simulink library "protectionLib"  (R2026a)
settings: Solver=VariableStepAuto
undefined symbols (not defined in the file or in its folder): DiscIntNeverNeededParam
settings Model: Creator=smred  LastModifiedBy=smred

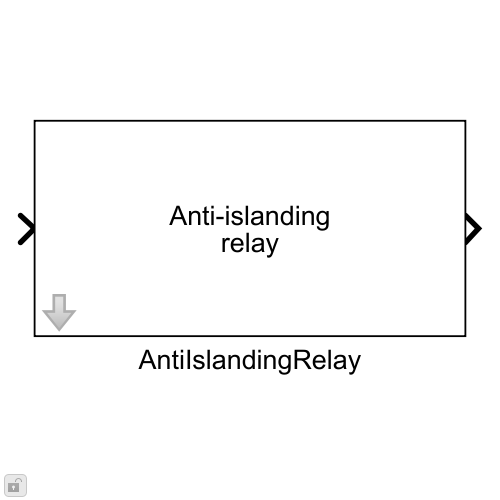
[thumbnail: Simulink's stored preview of the top-level diagram]
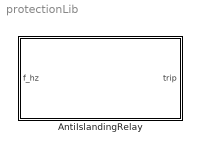
== system protectionLib ==
  AntiIslandingRelay : Subsystem  mask{f_min=47, f_max=52, t_arm=0.5, t_pickup=0.05, Ts=1e-4}
      mask prompts: f_min "Under-frequency trip (Hz)"; f_max "Over-frequency trip (Hz)"; t_arm "Relay blocked until (s)"; t_pickup "Out-of-band must persist (s)"; Ts "Persistence timer rate (s)"
      mask help:
      | Over/under-frequency relay with startup blocking and a persistence delay.
      |
      | Latches trip when the frequency estimate has been outside [f_min, f_max] continuously for t_pickup, and only after t_arm.
      |
      | BLOCKING (t_arm): a PLL frequency estimate is meaningless until the loop has acquired lock. Aqib's SRF-PLL leaves the 47-52 Hz band for up to 170 ms at startup, worst case at a 270 deg initial phase. Without blocking the relay latches at t = 0.
      |
      | PERSISTENCE (t_pickup): a 30 deg phase jump - the SC4 stimulus, which the PLL is specified to ride through - drives the estimate to 60 Hz for 12.4 ms, and a 60 deg jump for 20.7 ms. Without persistence the relay trips on a grid event the plant must survive. The default 50 ms gives 2.4x margin on the worst of those.
      |
      | Both figures are measured: see pll_startup_probe and pll_jump_probe.
      |
      | The latch is permanent. AS/NZS 4777.2 requires reconnection after 60 s within limits; that is not implemented here.
      mask Display: disp('Anti-islanding\nrelay')

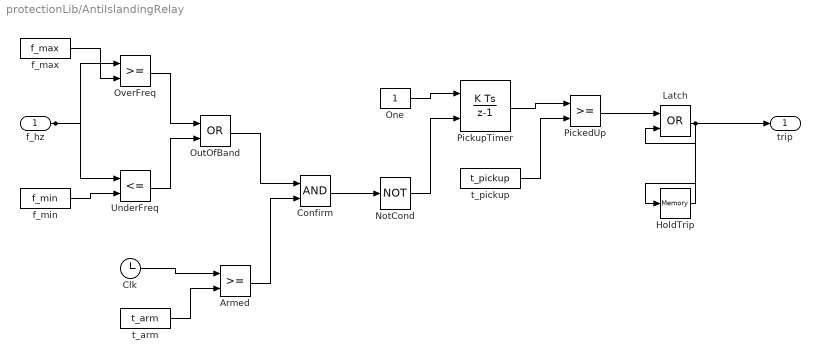
== system protectionLib/AntiIslandingRelay ==
  f_hz : Inport
  Armed : RelationalOperator  OutDataTypeStr=boolean  RndMeth=Simplest  InputSameDT=off
  Clk : Clock
  Confirm : Logic  AllPortsSameDT=off  OutDataTypeStr=boolean
  HoldTrip : Memory
  Latch : Logic  Operator=OR  AllPortsSameDT=off  OutDataTypeStr=boolean
  NotCond : Logic  Operator=NOT  Inputs=1  AllPortsSameDT=off  OutDataTypeStr=boolean
  One : Constant
  OutOfBand : Logic  Operator=OR  AllPortsSameDT=off  OutDataTypeStr=boolean
  OverFreq : RelationalOperator  OutDataTypeStr=boolean  RndMeth=Simplest  InputSameDT=off
  PickedUp : RelationalOperator  OutDataTypeStr=boolean  RndMeth=Simplest  InputSameDT=off
  PickupTimer : DiscreteIntegrator  gainval=1  ExternalReset=level  SampleTime=Ts  ICPrevOutput=DiscIntNeverNeededParam  ICPrevScaledInput=DiscIntNeverNeededParam
  UnderFreq : RelationalOperator  Operator=<=  OutDataTypeStr=boolean  RndMeth=Simplest  InputSameDT=off
  f_max : Constant  Value=f_max
  f_min : Constant  Value=f_min
  t_arm : Constant  Value=t_arm
  t_pickup : Constant  Value=t_pickup
  trip : Outport
  wires:
  f_hz/1 -> OverFreq/1, UnderFreq/1
  f_max/1 -> OverFreq/2
  f_min/1 -> UnderFreq/2
  OverFreq/1 -> OutOfBand/1
  UnderFreq/1 -> OutOfBand/2
  Clk/1 -> Armed/1
  t_arm/1 -> Armed/2
  OutOfBand/1 -> Confirm/1
  Armed/1 -> Confirm/2
  Confirm/1 -> NotCond/1
  One/1 -> PickupTimer/1
  NotCond/1 -> PickupTimer/2
  PickupTimer/1 -> PickedUp/1
  t_pickup/1 -> PickedUp/2
  PickedUp/1 -> Latch/1
  HoldTrip/1 -> Latch/2
  Latch/1 -> HoldTrip/1, trip/1
